simulink model "mainmodel"  (R2019b)
settings: Solver=VariableStepAuto  StartTime=0.0  StopTime=20  RelTol=1e-4
values from neighbouring files (symbols this model uses):
  flux = (60*56)/(2*3.14)    (= 535.031847134)    [model_initial.m]
  J = 0.0001279 + 5.51181*6.372e-7    (= 0.000131412125332)    [model_initial.m]
  Kicc = (currentloop_hz^2)*Ls    (= 117329.24)    [model_initial.m]
  Kipc = (positionloop_hz^2)    (= 985.96)    [model_initial.m]
  Kisc = (speedloop_hz^2)    (= 98596)    [model_initial.m]
  Kpcc = 2*(currentloop_hz*damping)/Ls - Rs    (= 373104.182353)    [model_initial.m]
  Kppc = 2*(positionloop_hz*damping)    (= 44.3996)    [model_initial.m]
  Kpsc = 2*(speedloop_hz*damping)*J    (= 0.0583464579989)    [model_initial.m]
  Ls = 11.9e-3    (= 0.0119)    [model_initial.m]
  polepair = 4    [model_initial.m]
  Rs = 1.7    [model_initial.m]
libraries: eeGeneralControl x2
settings Model: Creator=rafek  LastModifiedBy=rafek
settings SolverCC: ZeroCrossAlgorithm=Adaptive  AlgebraicLoopSolver=LineSearch
settings DebuggingCC: IgnoredZcDiagnostic=none

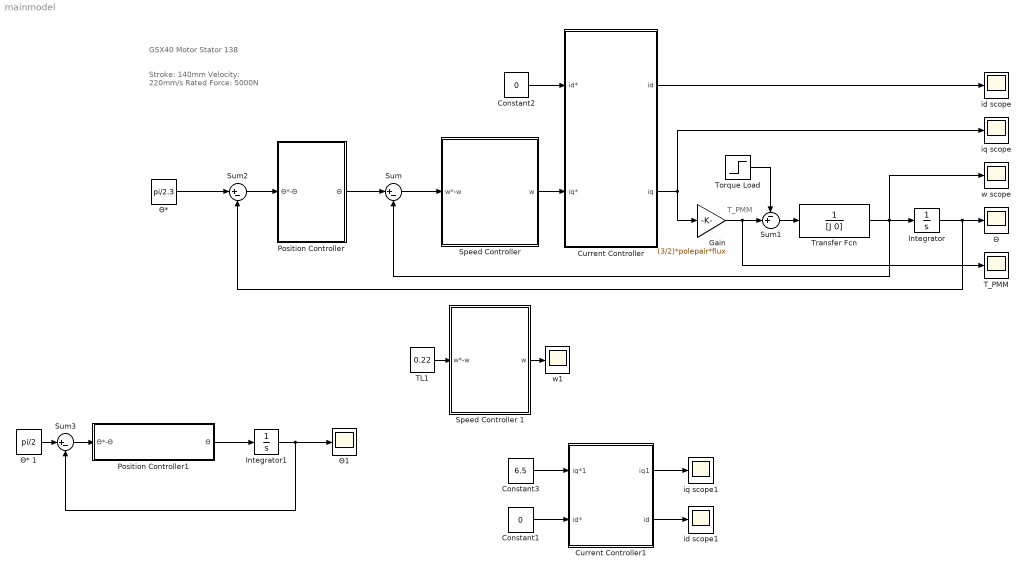
== system mainmodel ==
  note: T_PMM
  note: GSX40 Motor Stator 138
  note: Stroke: 140mm
      | Velocity: 220mm/s
      | Rated Force: 5000N
  Constant1 : Constant  Value=0
  Constant2 : Constant  Value=0
  Constant3 : Constant  Value=6.5
  Current Controller : Subsystem
  Current Controller1 : Subsystem
  "Gain " : Gain  Gain=(3/2)*polepair*flux
  Integrator : Integrator
  Integrator1 : Integrator
  Position Controller : Subsystem
  Position Controller1 : Subsystem
  "Speed Controller " : Subsystem
  Speed Controller 1 : Subsystem
  Sum : Sum  Inputs=|+-
  Sum1 : Sum  Inputs=-+|
  Sum2 : Sum  Inputs=|+-
  Sum3 : Sum  Inputs=|+-
  TL1 : Constant  Value=0.22
  T_PMM : Scope
  Torque Load : Step  Time=0  After=700  SampleTime=0
  Transfer Fcn : TransferFcn  Denominator=[J 0]
  id scope : Scope
  id scope1 : Scope
  iq scope : Scope
  iq scope1 : Scope
  w scope : Scope
  w1 : Scope
  Θ : Scope
  "Θ* " : Constant  Value=pi/2.3
  Θ* 1 : Constant  Value=pi/2
  Θ1 : Scope
  wires:
  Constant2/1 -> Current Controller/1(id*)
  Sum/1 -> "Speed Controller "/1(w*-w)
  Torque Load/1 -> Sum1/1
  "Gain "/1 -> Sum1/2, T_PMM/1
  Integrator/1 -> Θ/1, Sum2/2
  Current Controller/2("iq ") -> iq scope/1, "Gain "/1
  Position Controller/1(Θ) -> Sum/1
  Current Controller/1(id) -> id scope/1
  Current Controller1/1(iq1) -> iq scope1/1
  Constant1/1 -> Current Controller1/2(id*)
  Current Controller1/2(id) -> id scope1/1
  Constant3/1 -> Current Controller1/1(iq*1)
  Sum1/1 -> Transfer Fcn/1
  "Speed Controller "/1(w) -> Current Controller/2(iq*)
  Transfer Fcn/1 -> Integrator/1, w scope/1, Sum/2
  Speed Controller 1/1(w) -> w1/1
  TL1/1 -> Speed Controller 1/1(w*-w)
  "Θ* "/1 -> Sum2/1
  Integrator1/1 -> Sum3/2, Θ1/1
  Θ* 1/1 -> Sum3/1
  Sum3/1 -> Position Controller1/1(Θ*-Θ)
  Position Controller1/1(Θ) -> Integrator1/1
  Sum2/1 -> Position Controller/1(Θ*-Θ)

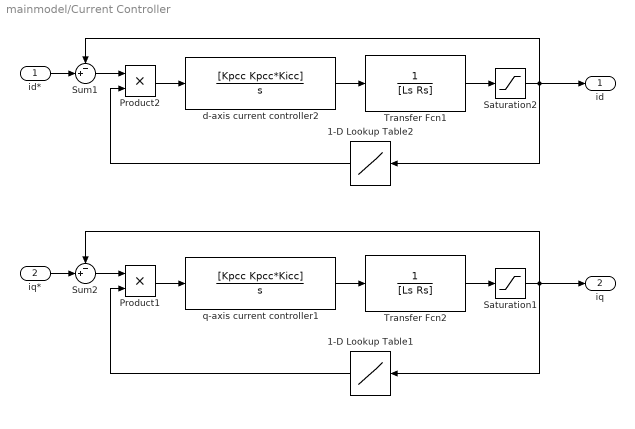
== system mainmodel/Current Controller ==
  id* : Inport
  iq* : Inport  Port=2
  1-D Lookup Table1 : Lookup_n-D  NumberOfTableDimensions=1  BreakpointsForDimension1=[-100, -6.6, -6.5, 0, 6.5, 6.6, 100]  Table=[0, 0, 1, 1, 1, 0, 0]  InternalRulePriority=Speed  RndMeth=Simplest  InputSameDT=on
  1-D Lookup Table2 : Lookup_n-D  NumberOfTableDimensions=1  BreakpointsForDimension1=[-100, -6.6, -6.5, 0, 6.5, 6.6, 100]  Table=[0, 0, 1, 1, 1, 0, 0]  InternalRulePriority=Speed  RndMeth=Simplest  InputSameDT=on
  Product1 : Product
  Product2 : Product
  Saturation1 : Saturate  UpperLimit=230  LowerLimit=-230
  Saturation2 : Saturate  UpperLimit=230  LowerLimit=-230
  Sum1 : Sum  Inputs=-+|
  Sum2 : Sum  Inputs=-+|
  Transfer Fcn1 : TransferFcn  Denominator=[Ls Rs]
  Transfer Fcn2 : TransferFcn  Denominator=[Ls Rs]
  d-axis current controller2 : TransferFcn  Numerator=[Kpcc Kpcc*Kicc]  Denominator=[1 0]
  q-axis current controller1 : TransferFcn  Numerator=[Kpcc Kpcc*Kicc]  Denominator=[1 0]
  id : Outport
  "iq " : Outport  Port=2
  wires:
  Transfer Fcn2/1 -> Saturation1/1
  Saturation1/1 -> 1-D Lookup Table1/1, Sum2/1, "iq "/1
  iq*/1 -> Sum2/2
  1-D Lookup Table1/1 -> Product1/2
  q-axis current controller1/1 -> Transfer Fcn2/1
  Product1/1 -> q-axis current controller1/1
  Sum2/1 -> Product1/1
  id*/1 -> Sum1/2
  Sum1/1 -> Product2/1
  Transfer Fcn1/1 -> Saturation2/1
  Saturation2/1 -> Sum1/1, 1-D Lookup Table2/1, id/1
  Product2/1 -> d-axis current controller2/1
  1-D Lookup Table2/1 -> Product2/2
  d-axis current controller2/1 -> Transfer Fcn1/1

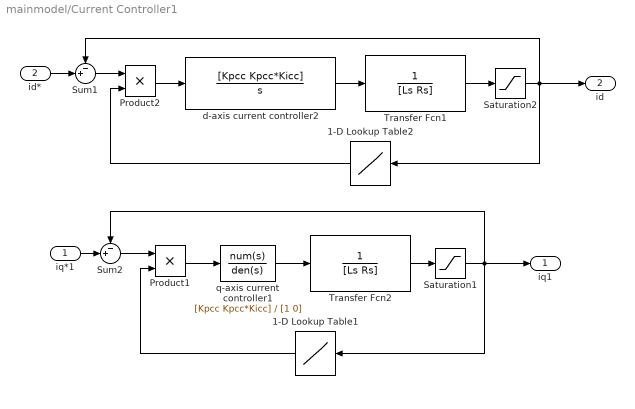
== system mainmodel/Current Controller1 ==
  iq*1 : Inport
  id* : Inport  Port=2
  1-D Lookup Table1 : Lookup_n-D  NumberOfTableDimensions=1  BreakpointsForDimension1=[-100, -6.6, -6.5, 0, 6.5, 6.6, 100]  Table=[0, 0, 1, 1, 1, 0, 0]  InternalRulePriority=Speed  RndMeth=Simplest  InputSameDT=on
  1-D Lookup Table2 : Lookup_n-D  NumberOfTableDimensions=1  BreakpointsForDimension1=[-100, -6.6, -6.5, 0, 6.5, 6.6, 100]  Table=[0, 0, 1, 1, 1, 0, 0]  InternalRulePriority=Speed  RndMeth=Simplest  InputSameDT=on
  Product1 : Product
  Product2 : Product
  Saturation1 : Saturate  UpperLimit=400  LowerLimit=-400
  Saturation2 : Saturate  UpperLimit=400  LowerLimit=-400
  Sum1 : Sum  Inputs=-+|
  Sum2 : Sum  Inputs=-+|
  Transfer Fcn1 : TransferFcn  Denominator=[Ls Rs]
  Transfer Fcn2 : TransferFcn  Denominator=[Ls Rs]
  d-axis current controller2 : TransferFcn  Numerator=[Kpcc Kpcc*Kicc]  Denominator=[1 0]
  q-axis current controller1 : TransferFcn  Numerator=[Kpcc Kpcc*Kicc]  Denominator=[1 0]
  iq1 : Outport
  id : Outport  Port=2
  wires:
  Transfer Fcn2/1 -> Saturation1/1
  Saturation1/1 -> 1-D Lookup Table1/1, Sum2/1, iq1/1
  iq*1/1 -> Sum2/2
  1-D Lookup Table1/1 -> Product1/2
  Sum2/1 -> Product1/1
  q-axis current controller1/1 -> Transfer Fcn2/1
  Product1/1 -> q-axis current controller1/1
  1-D Lookup Table2/1 -> Product2/2
  Saturation2/1 -> Sum1/1, 1-D Lookup Table2/1, id/1
  Product2/1 -> d-axis current controller2/1
  d-axis current controller2/1 -> Transfer Fcn1/1
  Sum1/1 -> Product2/1
  Transfer Fcn1/1 -> Saturation2/1
  id*/1 -> Sum1/2

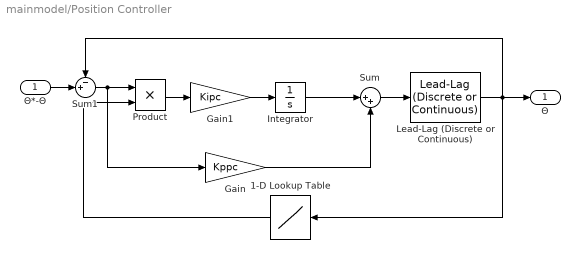
== system mainmodel/Position Controller ==
  Θ*-Θ : Inport
  1-D Lookup Table : Lookup_n-D  NumberOfTableDimensions=1  BreakpointsForDimension1=[-100, -0.23, -0.22, 0, 0.22, 0.23, 100]  Table=[0, 0, 1, 1, 1, 0, 0]  InternalRulePriority=Speed  RndMeth=Simplest  InputSameDT=on
  Gain : Gain  Gain=Kppc
  Gain1 : Gain  Gain=Kipc
  Integrator : Integrator
  Lead-Lag (Discrete or Continuous) : eeGeneralControl/Lead-Lag (Discrete or Continuous)  T1=1  T2=10*3.14  B=0.4  A=-0.4  Ts=0
      settings: SourceProductName=Simscape Electrical  SourceProductBaseCode=PS
  Product : Product
  Sum : Sum  Inputs=|++
  Sum1 : Sum  Inputs=-+|
  Θ : Outport
  wires:
  Lead-Lag (Discrete or Continuous)/1 -> Sum1/1, Θ/1, 1-D Lookup Table/1
  Gain1/1 -> Integrator/1
  Gain/1 -> Sum/2
  Integrator/1 -> Sum/1
  Sum/1 -> Lead-Lag (Discrete or Continuous)/1
  Sum1/1 -> Gain/1, Product/1
  Product/1 -> Gain1/1
  Θ*-Θ/1 -> Sum1/2
  1-D Lookup Table/1 -> Product/2

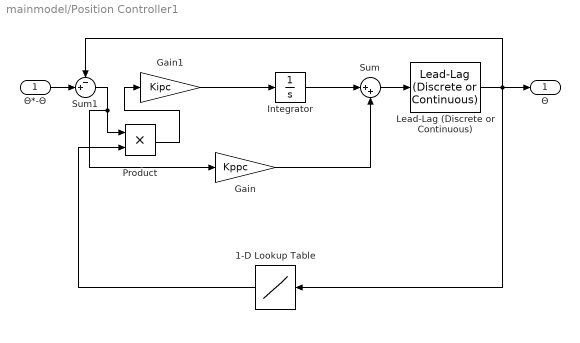
== system mainmodel/Position Controller1 ==
  Θ*-Θ : Inport
  1-D Lookup Table : Lookup_n-D  NumberOfTableDimensions=1  BreakpointsForDimension1=[-100, -0.22, -0.21, 0, 0.21, 0.22, 100]  Table=[0, 0, 1, 1, 1, 0, 0]  InternalRulePriority=Speed  RndMeth=Simplest  InputSameDT=on
  Gain : Gain  Gain=Kppc
  Gain1 : Gain  Gain=Kipc
  Integrator : Integrator
  Lead-Lag (Discrete or Continuous) : eeGeneralControl/Lead-Lag (Discrete or Continuous)  T1=1  T2=10*3.14  B=220  A=-220  Ts=0
      settings: SourceProductName=Simscape Electrical  SourceProductBaseCode=PS
  Product : Product
  Sum : Sum  Inputs=|++
  Sum1 : Sum  Inputs=-+|
  Θ : Outport
  wires:
  Gain1/1 -> Integrator/1
  Gain/1 -> Sum/2
  Integrator/1 -> Sum/1
  Sum/1 -> Lead-Lag (Discrete or Continuous)/1
  Sum1/1 -> Product/1, Gain/1
  1-D Lookup Table/1 -> Product/2
  Lead-Lag (Discrete or Continuous)/1 -> Sum1/1, 1-D Lookup Table/1, Θ/1
  Θ*-Θ/1 -> Sum1/2
  Product/1 -> Gain1/1

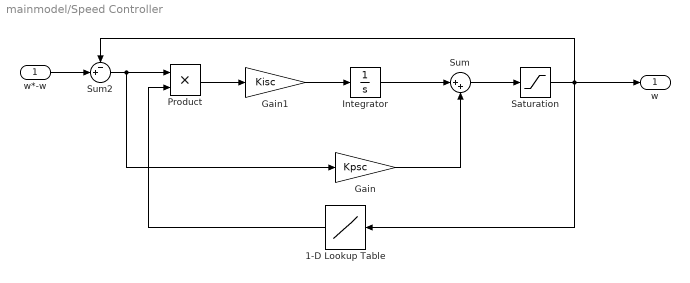
== system mainmodel/Speed Controller  ==
  w*-w : Inport
  1-D Lookup Table : Lookup_n-D  NumberOfTableDimensions=1  BreakpointsForDimension1=[-100, -0.22, -0.21, 0, 0.21, 0.22, 100]  Table=[0, 0, 1, 1, 1, 0, 0]  InternalRulePriority=Speed  RndMeth=Simplest  InputSameDT=on
  Gain : Gain  Gain=Kpsc
  Gain1 : Gain  Gain=Kisc
  Integrator : Integrator
  Product : Product
  Saturation : Saturate  UpperLimit=9.1  LowerLimit=-9.1
  Sum : Sum  Inputs=|++
  Sum2 : Sum  Inputs=-+|
  w : Outport
  wires:
  Gain1/1 -> Integrator/1
  Gain/1 -> Sum/2
  Integrator/1 -> Sum/1
  w*-w/1 -> Sum2/2
  Sum2/1 -> Gain/1, Product/1
  Product/1 -> Gain1/1
  1-D Lookup Table/1 -> Product/2
  Sum/1 -> Saturation/1
  Saturation/1 -> 1-D Lookup Table/1, w/1, Sum2/1

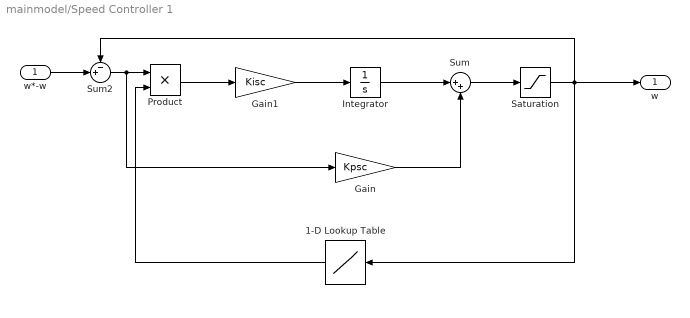
== system mainmodel/Speed Controller 1 ==
  w*-w : Inport
  1-D Lookup Table : Lookup_n-D  NumberOfTableDimensions=1  BreakpointsForDimension1=[-100, -0.22, -0.21, 0, 0.21, 0.22, 100]  Table=[0, 0, 1, 1, 1, 0, 0]  InternalRulePriority=Speed  RndMeth=Simplest  InputSameDT=on
  Gain : Gain  Gain=Kpsc
  Gain1 : Gain  Gain=Kisc
  Integrator : Integrator
  Product : Product
  Saturation : Saturate  UpperLimit=9.1  LowerLimit=-9.1
  Sum : Sum  Inputs=|++
  Sum2 : Sum  Inputs=-+|
  w : Outport
  wires:
  Gain1/1 -> Integrator/1
  Gain/1 -> Sum/2
  Integrator/1 -> Sum/1
  w*-w/1 -> Sum2/2
  Sum2/1 -> Gain/1, Product/1
  Product/1 -> Gain1/1
  1-D Lookup Table/1 -> Product/2
  Sum/1 -> Saturation/1
  Saturation/1 -> 1-D Lookup Table/1, w/1, Sum2/1
